simulink model "verify_Date2Sec_mdl"  (R2016b)
settings: Solver=ode45  StartTime=0  StopTime=24*3600+1  MaxStep=1800  RelTol=1e-3  EnableMultiTasking=on
libraries: carnot x2
settings Model: Creator=drhf  LastModifiedBy=drhf
settings DataIOCC: SaveFormat=Array  SignalLoggingSaveFormat=ModelDataLogs
settings OptimizationCC: ExpressionDepthLimit=2147483647  LifeSpan=inf
settings DebuggingCC: UnderspecifiedInitializationDetection=Classic  MergeDetectMultiDrivingBlocksExec=none  SolverPrmCheckMsg=warning  FcnCallInpInsideContextMsg=warning  StateNameClashWarn=warning  SFUnexpectedBacktrackingDiag=warning  SFNoUnconditionalDefaultTransitionDiag=warning  SFExecutionAtInitializationDiag=none
settings HardwareCC: ProdBitPerPointer=32  ProdBitPerSizeT=32  ProdBitPerPtrDiffT=32  ProdLargestAtomicFloat=None  ProdIntDivRoundTo=Undefined  ProdEndianess=Unspecified  ProdWordSize=32  ProdHWDeviceType=32-bit Generic
settings ModelReferenceCC: PropagateSignalLabelsOutOfModel=off
settings GRTTargetCC: TargetLangStandard=C89/C90 (ANSI)  GeneratePreprocessorConditionals=Disable all  CombineOutputUpdateFcns=off  GRTInterface=on
settings ConfigComp: CovMetricSettings=dw  CovHtmlReporting=on  CovSaveCumulativeToWorkspaceVar=on  CovSaveSingleToWorkspaceVar=on  CovExternalEMLEnable=off

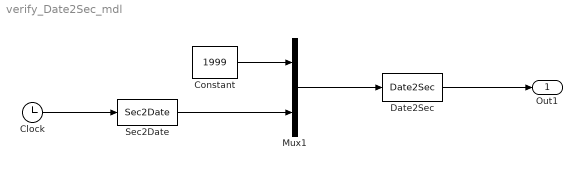
== system verify_Date2Sec_mdl ==
  Clock : Clock
  Constant : Constant  Value=1999
  Date2Sec : carnot/Toolbox/Date2Sec
  Mux1 : Mux  Inputs=2
  Sec2Date : carnot/Toolbox/Sec2Date
  Out1 : Outport
  wires:
  Date2Sec/1 -> Out1/1
  Clock/1 -> Sec2Date/1
  Sec2Date/1 -> Mux1/2
  Constant/1 -> Mux1/1
  Mux1/1 -> Date2Sec/1
